simulink model "sampleModel1738"  (R2023a)
settings: Solver=VariableStepAuto  StartTime=0.0  StopTime=10.0  RelTol=1e-3
libraries: hdlsllib x3, simulink x2
settings Model: Creator=user1  LastModifiedBy=user1

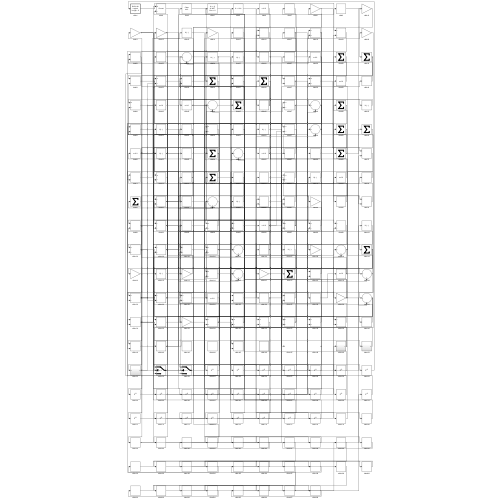
[thumbnail: Simulink's stored preview of the top-level diagram]
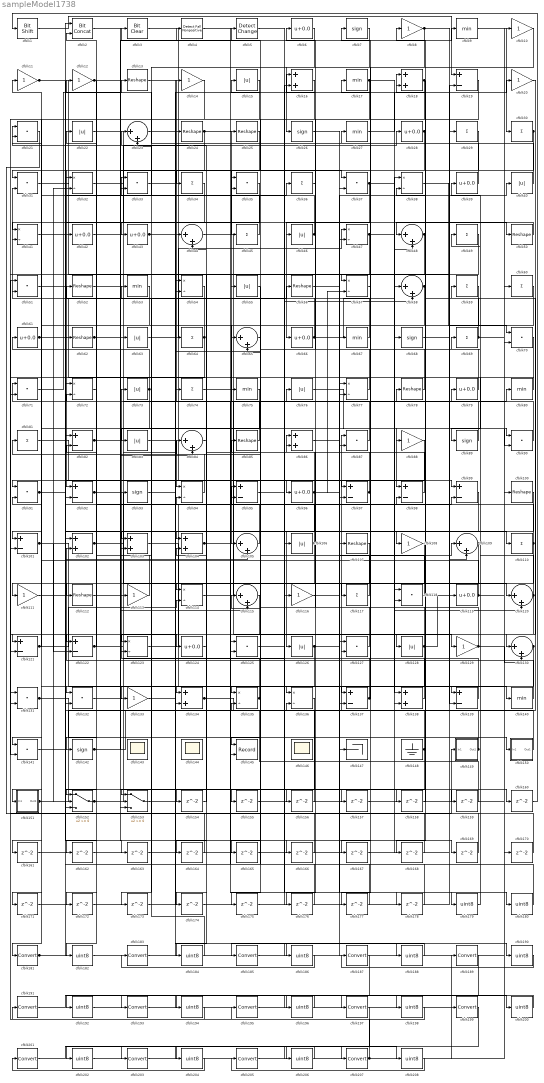
== system sampleModel1738 ==
  cfblk1 : hdlsllib/Logic and Bit Operations/Bit Shift  mode=Shift Left Logical  N=0
  cfblk{8,10..12,14,20,88,108,111,113,116,129,133} (13 alike) : Gain
  cfblk{13,24..25,50,52,56,62,78,85,100,107,112} (12 alike) : Reshape
  cfblk{19,82,92,95,97..99,101,121..122,137,139} (12 alike) : Sum  Inputs=+-
  cfblk{16,18,86,102..104,134,138} (8 alike) : Sum
  cfblk{23,44,48,58,65,84,105,109,115,120,130} (11 alike) : Sum  Inputs=|++
  cfblk{15,22,40,46,55,63,73,76,83,106,126,128} (12 alike) : Abs  SaturateOnIntegerOverflow=off
  cfblk{29..30,34,36,45,49,59..60,64,69,74,81,110,117} (14 alike) : Sum  Inputs=+
  cfblk{32,38,41,47,54,57,72,77,94,114,123,135..136} (13 alike) : Product  Inputs=*/  RndMeth=Zero  SaturateOnIntegerOverflow=on
  cfblk{21,31,33,35,37,51,70..71,87,90..91,118,125,127,131..132,141} (17 alike) : DotProduct  OutDataTypeStr=Inherit: Inherit via internal rule
  cfblk{6,28,39,42..43,61,66,79,96,119,124} (11 alike) : Bias  Bias=0.0  SaturateOnIntegerOverflow=off
  cfblk{9,17,27,53,67,75,80,140} (8 alike) : MinMax
  cfblk{7,26,68,89,93,142} (6 alike) : Signum
  cfblk143 : Scope
      settings: Floating=on
  cfblk144 : Scope
      settings: Floating=on
  cfblk145 : Record  FileSettingsInternal="{\"entries\":[{\"content\":{\"excelSettings\":{\"content\":{},\"type\":\"Streamout.ExcelSettings\"}},\"type\":\"Streamout.FileSettingStorage\",\"uuid\":\"\"}],\"packageUris\":[\"http:\\/\\/schema.mathworks.com\\/mf0\\/streamout_blocks\\/R2020a\"],\"version\":\"1.0\"}"  Layout=[1 1]  SignalsInternal="{\"entries\":[{\"content\":{\"signals\":[{\"content\":{\"blockPath\":[],\"dimensions\":[1],\"domain\":\"\",\"lineColor\":\"#a2142f\",\"plots\":[1],\"port\":1,\"signalID\":3516,\"signalName\":\"XY Graph:1\"},\"type\":\"RecordBlkView.Signal\",\"uuid\":\"\"},{\"content\":{\"blockPath\":[],\"dimensions\":[1],\"domain\":\"\",\"lineColor\":\"#139fff\",\"plots\":[1],\"port\":2,\"signalID\":3519,\"signalName\":\"XY Graph:2\"},\"type\":\"RecordBlkView.Signal\",\"uuid\":\"\"}]},\"type\":\"RecordBlkView.InputSignals\",\"uuid\":\"\"}],\"packageUris\":[\"http:\\/\\/schema.mathworks.com\\/mf0\\/streamout_blocks\\/R2020a\"],\"version\":\"1.0\"}"  VisualizationBindings="{\"xyplotplugin\":{\"info\":[{\"series\":[{\"bindingParametersList\":[{\"parameter\":\"X-Axis\",\"signalID\":3516,\"signalName\":\"XY Graph:1\"},{\"parameter\":\"Y-Axis\",\"signalID\":3519,\"signalName\":\"XY Graph:2\"}],\"seriesID\":43159}],\"subplotID\":1}]}}"  CompatibilityTag=XY  st=-1
  cfblk146 : Scope
      settings: Floating=on
  cfblk147 : Terminator
  cfblk148 : Ground
  cfblk149 : Subsystem
      settings: LibrarySourceBlock=|
      | hdlsllib/Ports &
      | Subsystems/Subsystem
  cfblk150 : Subsystem
      settings: LibrarySourceBlock=|
      | hdlsllib/Ports &
      | Subsystems/Subsystem
  cfblk151 : Subsystem
      settings: LibrarySourceBlock=|
      | hdlsllib/Ports &
      | Subsystems/Subsystem
  cfblk152 : Switch  SaturateOnIntegerOverflow=off  InputSameDT=off
  cfblk153 : Switch  SaturateOnIntegerOverflow=off  InputSameDT=off
  cfblk{154..178} (25 alike) : Delay  SampleTime=1
  cfblk{179..180,182,184,186,188,190,192,194,196,198,200,202,204,206,208} (16 alike) : DataTypeConversion  OutDataTypeStr=uint8  SaturateOnIntegerOverflow=off  RndMeth=Floor
  cfblk{181,183,185,187,189,191,193,195,197,199,201,203,205,207} (14 alike) : DataTypeConversion  SaturateOnIntegerOverflow=off  RndMeth=Floor
  cfblk2 : hdlsllib/Logic and Bit Operations/Bit Concat  numInputs=2
  cfblk3 : simulink/Logic and Bit Operations/Bit Clear  iBit=0
      settings: LibrarySourceBlock=|
      | hdlsllib/Logic and Bit
      | Operations/Bit Clear
  cfblk4 : hdlsllib/Logic and Bit Operations/Detect Fall Nonpositive  vinit=0  OutDataTypeStr=boolean
  cfblk5 : simulink/Logic and Bit Operations/Detect Change  vinit=0  OutDataTypeStr=boolean
      settings: LibrarySourceBlock=|
      | hdlsllib/Logic and Bit
      | Operations/Detect
      | Change
  wires:
  cfblk8/1 -> cfblk26/1, cfblk90/2
  cfblk114/1 -> cfblk80/1
  cfblk82/1 -> cfblk28/1, cfblk88/1, cfblk139/1
  cfblk87/1 -> cfblk71/1
  cfblk130/1 -> cfblk132/1, cfblk172/1, cfblk173/1
  cfblk135/1 -> cfblk73/1, cfblk65/1
  cfblk134/1 -> cfblk59/1, cfblk44/2
  cfblk105/1 -> cfblk53/1
  cfblk53/1 -> cfblk92/1
  cfblk131/1 -> cfblk36/1, cfblk105/2, cfblk150/1(In1)
  cfblk150/1(Out1) -> cfblk87/1
  cfblk38/1 -> cfblk70/1
  cfblk1/1 -> cfblk19/1
  cfblk101/1 -> cfblk135/1, cfblk122/2
  cfblk71/1 -> cfblk13/1
  cfblk74/1 -> cfblk97/1
  cfblk50/1 -> cfblk48/1
  cfblk132/1 -> cfblk25/1
  cfblk73/1 -> cfblk61/1, cfblk92/2
  cfblk142/1 -> cfblk63/1, cfblk67/1
  cfblk100/1 -> cfblk126/1
  cfblk63/1 -> cfblk47/1
  cfblk137/1 -> cfblk27/1, cfblk115/1
  cfblk11/1 -> cfblk57/1, cfblk99/1, cfblk50/1
  cfblk37/1 -> cfblk66/1, cfblk90/1
  cfblk66/1 -> cfblk136/1, cfblk48/2, cfblk41/2
  cfblk83/1 -> cfblk94/1
  cfblk39/1 -> cfblk12/1
  cfblk43/1 -> cfblk127/1, cfblk139/2
  cfblk18/1 -> cfblk108/1, cfblk101/1
  cfblk79/1 -> cfblk3/1
  cfblk122/1 -> cfblk94/2, cfblk82/2
  cfblk36/1 -> cfblk96/1
  cfblk92/1 -> cfblk120/1, cfblk166/1
  cfblk128/1 -> cfblk119/1, cfblk137/2, cfblk86/2
  cfblk7/1 -> cfblk123/1
  cfblk151/1(Out1) -> cfblk47/2, cfblk32/2
  cfblk44/1 -> cfblk129/1
  cfblk17/1 -> cfblk120/2, cfblk23/2, cfblk176/1
  cfblk102/1 -> cfblk79/1, cfblk98/2
  cfblk91/1 -> cfblk56/1, cfblk99/2
  cfblk116/1 -> cfblk147/1
  cfblk3/1 -> cfblk138/1
  cfblk75/1 -> cfblk141/1
  cfblk25/1 -> cfblk72/1
  cfblk148/1 -> cfblk136/2, cfblk153/1
  cfblk59/1 -> cfblk105/1
  cfblk152/1 -> cfblk106/1, cfblk153/2
  cfblk24/1 -> cfblk31/1, cfblk159/1
  cfblk9/1 -> cfblk30/1
  cfblk85/1 -> cfblk14/1
  cfblk123/1 -> cfblk95/1
  cfblk153/1 -> cfblk24/1
  cfblk90/1 -> cfblk15/1
  cfblk69/1 -> cfblk10/1, cfblk8/1
  cfblk94/1 -> cfblk52/1
  cfblk45/1 -> cfblk11/1
  cfblk126/1 -> cfblk109/1, cfblk151/1(In1)
  cfblk67/1 -> cfblk31/2
  cfblk109/1 -> cfblk125/2, cfblk69/1
  cfblk120/1 -> cfblk141/2, cfblk76/1
  cfblk23/1 -> cfblk117/1
  cfblk111/1 -> cfblk32/1
  cfblk129/1 -> cfblk4/1, cfblk130/2, cfblk49/1, cfblk64/1
  cfblk106/1 -> cfblk85/1, cfblk161/1
  cfblk119/1 -> cfblk100/1, cfblk21/2, cfblk111/1
  cfblk6/1 -> cfblk43/1
  cfblk80/1 -> cfblk75/1
  cfblk21/1 -> cfblk149/1(In1)
  cfblk95/1 -> cfblk128/1
  cfblk28/1 -> cfblk45/1, cfblk168/1
  cfblk47/1 -> cfblk118/1, cfblk184/1
  cfblk125/1 -> cfblk58/2
  cfblk103/1 -> cfblk140/1
  cfblk27/1 -> cfblk20/1
  cfblk88/1 -> cfblk133/1
  cfblk19/1 -> cfblk35/1
  cfblk16/1 -> cfblk131/2
  cfblk139/1 -> cfblk127/2
  cfblk15/1 -> cfblk83/1
  cfblk96/1 -> cfblk104/1, cfblk57/2, cfblk51/2, cfblk40/1
  cfblk2/1 -> cfblk37/1
  cfblk34/1 -> cfblk41/1
  cfblk113/1 -> cfblk2/2
  cfblk77/1 -> cfblk16/1
  cfblk31/1 -> cfblk107/1
  cfblk107/1 -> cfblk114/1
  cfblk48/1 -> cfblk71/2, cfblk121/2
  cfblk104/1 -> cfblk78/1, cfblk180/1
  cfblk60/1 -> cfblk181/1
  cfblk98/1 -> cfblk21/1
  cfblk30/1 -> cfblk34/1, cfblk37/2
  cfblk51/1 -> cfblk110/1
  cfblk117/1 -> cfblk72/2
  cfblk20/1 -> cfblk130/1
  cfblk32/1 -> cfblk46/1
  cfblk140/1 -> cfblk102/2
  cfblk149/1(Out1) -> cfblk84/1, cfblk65/2
  cfblk81/1 -> cfblk116/1
  cfblk33/1 -> cfblk18/1
  cfblk138/1 -> cfblk7/1
  cfblk70/1 -> cfblk89/1
  cfblk22/1 -> cfblk68/1
  cfblk127/1 -> cfblk81/1
  cfblk12/1 -> cfblk142/1, cfblk115/2
  cfblk112/1 -> cfblk54/2
  cfblk76/1 -> cfblk98/1
  cfblk35/1 -> cfblk112/1
  cfblk58/1 -> cfblk38/2, cfblk121/1
  cfblk110/1 -> cfblk22/1, cfblk134/1, cfblk152/3, cfblk175/1
  cfblk118/1 -> cfblk33/1
  cfblk46/1 -> cfblk23/1, cfblk33/2
  cfblk121/1 -> cfblk114/2, cfblk42/1, cfblk153/3, cfblk91/2
  cfblk49/1 -> cfblk82/1
  cfblk78/1 -> cfblk6/1
  cfblk64/1 -> cfblk152/1, cfblk62/1, cfblk101/2
  cfblk54/1 -> cfblk103/1
  cfblk52/1 -> cfblk84/2
  cfblk61/1 -> cfblk55/1, cfblk113/1, cfblk145/2
  cfblk115/1 -> cfblk122/1
  cfblk4/1 -> cfblk137/1
  cfblk55/1 -> cfblk145/1
  cfblk99/1 -> cfblk152/2
  cfblk86/1 -> cfblk77/2
  cfblk89/1 -> cfblk74/1
  cfblk40/1 -> cfblk17/1
  cfblk97/1 -> cfblk86/1, cfblk91/1
  cfblk68/1 -> cfblk29/1
  cfblk62/1 -> cfblk9/1, cfblk124/1
  cfblk108/1 -> cfblk154/1
  cfblk154/1 -> cfblk104/2
  cfblk136/1 -> cfblk155/1
  cfblk155/1 -> cfblk58/1
  cfblk13/1 -> cfblk156/1
  cfblk156/1 -> cfblk2/1
  cfblk141/1 -> cfblk157/1
  cfblk157/1 -> cfblk70/2
  cfblk42/1 -> cfblk158/1
  cfblk158/1 -> cfblk18/2
  cfblk159/1 -> cfblk135/2
  cfblk56/1 -> cfblk160/1
  cfblk160/1 -> cfblk1/1
  cfblk161/1 -> cfblk19/2
  cfblk72/1 -> cfblk162/1
  cfblk162/1 -> cfblk95/2
  cfblk41/1 -> cfblk163/1
  cfblk163/1 -> cfblk138/2
  cfblk84/1 -> cfblk164/1
  cfblk164/1 -> cfblk131/1
  cfblk65/1 -> cfblk165/1
  cfblk165/1 -> cfblk118/2
  cfblk166/1 -> cfblk123/2
  cfblk57/1 -> cfblk167/1
  cfblk167/1 -> cfblk38/1
  cfblk168/1 -> cfblk103/2
  cfblk133/1 -> cfblk169/1
  cfblk169/1 -> cfblk77/1
  cfblk170/1 -> cfblk54/1
  cfblk29/1 -> cfblk171/1
  cfblk171/1 -> cfblk97/2
  cfblk172/1 -> cfblk134/2
  cfblk173/1 -> cfblk44/1
  cfblk124/1 -> cfblk174/1
  cfblk174/1 -> cfblk16/2
  cfblk175/1 -> cfblk109/2
  cfblk176/1 -> cfblk125/1
  cfblk10/1 -> cfblk177/1
  cfblk177/1 -> cfblk35/2
  cfblk26/1 -> cfblk178/1
  cfblk178/1 -> cfblk102/1
  cfblk5/1 -> cfblk179/1
  cfblk179/1 -> cfblk39/1
  cfblk180/1 -> cfblk5/1
  cfblk181/1 -> cfblk132/2, cfblk87/2
  cfblk14/1 -> cfblk182/1
  cfblk182/1 -> cfblk60/1
  cfblk184/1 -> cfblk93/1
  cfblk93/1 -> cfblk186/1
  cfblk186/1 -> cfblk183/1
  cfblk183/1 -> cfblk188/1
  cfblk188/1 -> cfblk185/1
  cfblk185/1 -> cfblk190/1
  cfblk190/1 -> cfblk187/1
  cfblk187/1 -> cfblk192/1
  cfblk192/1 -> cfblk189/1
  cfblk189/1 -> cfblk194/1
  cfblk194/1 -> cfblk191/1
  cfblk191/1 -> cfblk196/1
  cfblk196/1 -> cfblk193/1
  cfblk193/1 -> cfblk198/1
  cfblk198/1 -> cfblk195/1
  cfblk195/1 -> cfblk200/1
  cfblk200/1 -> cfblk197/1
  cfblk197/1 -> cfblk202/1
  cfblk202/1 -> cfblk199/1
  cfblk199/1 -> cfblk204/1
  cfblk204/1 -> cfblk201/1
  cfblk205/1 -> cfblk207/1
  cfblk201/1 -> cfblk206/1
  cfblk206/1 -> cfblk203/1
  cfblk207/1 -> cfblk170/1, cfblk51/1
  cfblk203/1 -> cfblk208/1
  cfblk208/1 -> cfblk205/1

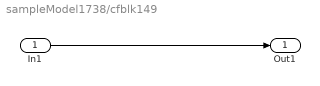
== system sampleModel1738/cfblk149 ==
  In1 : Inport
  Out1 : Outport
  wires:
  In1/1 -> Out1/1

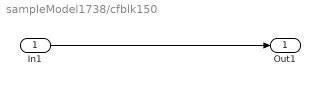
== system sampleModel1738/cfblk150 ==
  In1 : Inport
  Out1 : Outport
  wires:
  In1/1 -> Out1/1

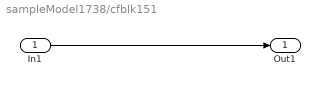
== system sampleModel1738/cfblk151 ==
  In1 : Inport
  Out1 : Outport
  wires:
  In1/1 -> Out1/1
